simulink model "ex3_3a"  (R2020a)
settings: Solver=VariableStepDiscrete  StartTime=-pi  StopTime=pi  RelTol=1e-3
libraries: simulink x1
settings Model: Creator=반달  LastModifiedBy=반달

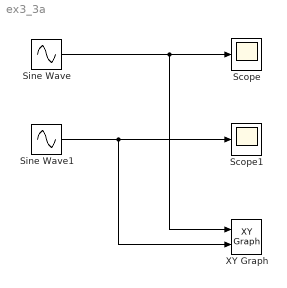
== system ex3_3a ==
  Scope : Scope
  Scope1 : Scope
  Sine Wave : Sin  Amplitude=10  Phase=pi/2  SampleTime=0.01
  Sine Wave1 : Sin  Amplitude=10  SampleTime=0.01
  XY Graph : simulink/Sinks/XY Graph  xmin=-10  xmax=10  ymin=-10  ymax=10  st=-1
  wires:
  Sine Wave/1 -> Scope/1, XY Graph/1
  Sine Wave1/1 -> XY Graph/2, Scope1/1
